simulink model "lab1"  (R2022b)
settings: Solver=VariableStepAuto  StartTime=0.0  StopTime=10.0  RelTol=1e-3
settings Model: Creator=dambi  LastModifiedBy=dambi

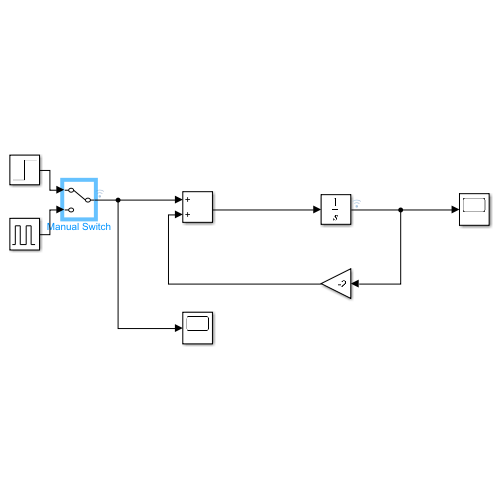
[thumbnail: Simulink's stored preview of the top-level diagram]
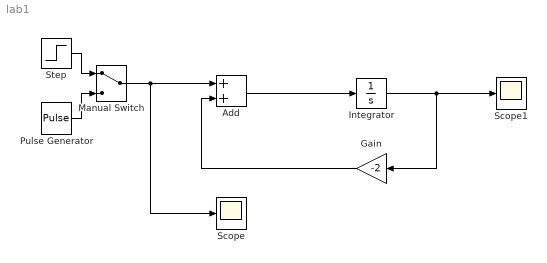
== system lab1 ==
  Add : Sum
  Gain : Gain  Gain=-2
  Integrator : Integrator
  Manual Switch : ManualSwitch
  Pulse Generator : DiscretePulseGenerator  PulseType=Time based  PulseWidth=20
  Scope : Scope
  Scope1 : Scope
  Step : Step  Time=2  SampleTime=0
  wires:
  Pulse Generator/1 -> Manual Switch/2
  Step/1 -> Manual Switch/1
  Manual Switch/1 -> Scope/1, Add/1
  Add/1 -> Integrator/1
  Integrator/1 -> Gain/1, Scope1/1
  Gain/1 -> Add/2
